simulink model "Clock_Model"  (R2025a)
settings: Solver=VariableStepAuto  StartTime=0.0  StopTime=1000  RelTol=1e-3
libraries: simulink_extras x27
(part 1 of 2)
settings Model: Creator=User  LastModifiedBy=User

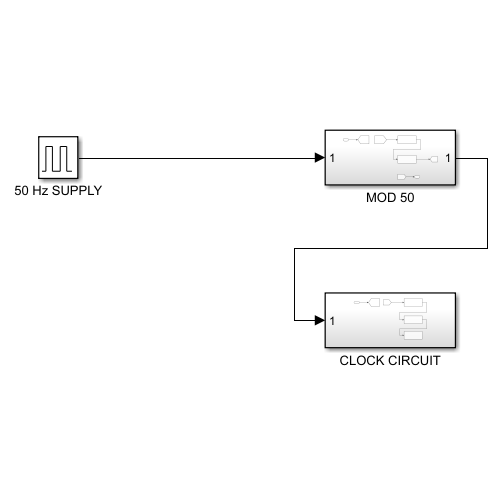
[thumbnail: Simulink's stored preview of the top-level diagram]
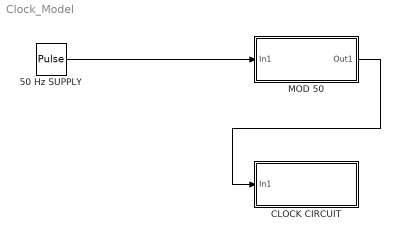
== system Clock_Model ==
  50 Hz SUPPLY : DiscretePulseGenerator  PulseType=Time based  Period=0.02  PulseWidth=50
  CLOCK CIRCUIT : Subsystem
  MOD 50 : Subsystem
  wires:
  50 Hz SUPPLY/1 -> MOD 50/1(In1)
  MOD 50/1(Out1) -> CLOCK CIRCUIT/1(In1)

== system Clock_Model/CLOCK CIRCUIT ==
  In1 : Inport
  HOURS : Subsystem
  MINUTES : Subsystem
  SECONDS : Subsystem
  wires:
  [Supply] -> SECONDS/1(In1)
  In1/1 -> [Supply]
  SECONDS/1(Out1) -> MINUTES/1(In2)
  MINUTES/1(Out1) -> HOURS/1(In1)

== system Clock_Model/MOD 50 ==
  In1 : Inport
  MOD 10 : Subsystem
  MOD 5 : Subsystem
  Out1 : Outport
  wires:
  In1/1 -> [Supply]
  MOD 10/1(Out1) -> MOD 5/1(In2)
  MOD 5/1(Out1) -> [Pulse]
  [Pulse] -> Out1/1
  [Supply] -> MOD 10/1(In1)

== system Clock_Model/CLOCK CIRCUIT/HOURS ==
  In1 : Inport
  MOD 13 : Subsystem
  wires:
  In1/1 -> MOD 13/1(In2)

== system Clock_Model/CLOCK CIRCUIT/MINUTES ==
  In2 : Inport
  MOD 60 : Subsystem
  Out1 : Outport
  wires:
  In2/1 -> MOD 60/1(In2)
  MOD 60/1(Out1) -> Out1/1

== system Clock_Model/CLOCK CIRCUIT/SECONDS ==
  In1 : Inport
  MOD 60 : Subsystem
  Out1 : Outport
  wires:
  In1/1 -> MOD 60/1(In2)
  MOD 60/1(Out1) -> Out1/1

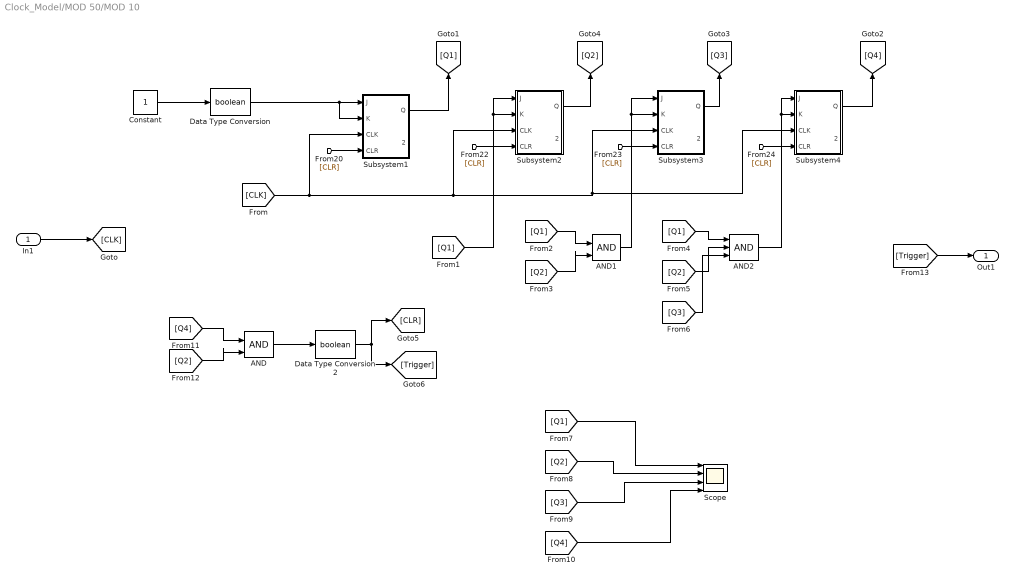
== system Clock_Model/MOD 50/MOD 10 ==
  In1 : Inport
  AND : Logic  IconShape=distinctive  AllPortsSameDT=off  OutDataTypeStr=boolean
  AND1 : Logic  IconShape=distinctive  AllPortsSameDT=off  OutDataTypeStr=boolean
  AND2 : Logic  Inputs=3  IconShape=distinctive  AllPortsSameDT=off  OutDataTypeStr=boolean
  Constant : Constant
  Data Type Conversion : DataTypeConversion  OutDataTypeStr=boolean  SaturateOnIntegerOverflow=off  RndMeth=Floor
  Data Type Conversion2 : DataTypeConversion  OutDataTypeStr=boolean  SaturateOnIntegerOverflow=off  RndMeth=Floor
  Scope : Scope  NumInputPorts=4
      settings: ActiveDisplayYMinimum=-1  ActiveDisplayYMaximum=1
  Subsystem1 : Subsystem
  Subsystem2 : Subsystem
  Subsystem3 : Subsystem
  Subsystem4 : Subsystem
  Out1 : Outport
  wires:
  [CLR] -> Subsystem2/4(CLR)
  [CLK] -> Subsystem1/3(CLK), Subsystem2/3(CLK), Subsystem4/3(CLK), Subsystem3/3(CLK)
  Data Type Conversion/1 -> Subsystem1/2(K), Subsystem1/1(J)
  [Q1] -> AND1/1
  AND1/1 -> Subsystem3/2(K), Subsystem3/1(J)
  [CLR] -> Subsystem1/4(CLR)
  [Q4] -> AND/1
  [Q2] -> AND2/2
  [Q1] -> AND2/1
  Subsystem1/1(Q) -> [Q1]
  [Q3] -> AND2/3
  [Q2] -> AND1/2
  Constant/1 -> Data Type Conversion/1
  AND2/1 -> Subsystem4/2(K), Subsystem4/1(J)
  Subsystem4/1(Q) -> [Q4]
  [CLR] -> Subsystem4/4(CLR)
  [Q1] -> Subsystem2/2(K), Subsystem2/1(J)
  [Q2] -> AND/2
  Subsystem2/1(Q) -> [Q2]
  Data Type Conversion2/1 -> [CLR], [Trigger]
  [CLR] -> Subsystem3/4(CLR)
  Subsystem3/1(Q) -> [Q3]
  AND/1 -> Data Type Conversion2/1
  In1/1 -> [CLK]
  [Trigger] -> Out1/1
  [Q1] -> Scope/1
  [Q2] -> Scope/2
  [Q3] -> Scope/3
  [Q4] -> Scope/4

== system Clock_Model/MOD 50/MOD 5 ==
  In2 : Inport
  AND : Logic  IconShape=distinctive  AllPortsSameDT=off  OutDataTypeStr=boolean
  AND1 : Logic  IconShape=distinctive  AllPortsSameDT=off  OutDataTypeStr=boolean
  Constant : Constant
  Data Type Conversion : DataTypeConversion  OutDataTypeStr=boolean  SaturateOnIntegerOverflow=off  RndMeth=Floor
  Data Type Conversion2 : DataTypeConversion  OutDataTypeStr=boolean  SaturateOnIntegerOverflow=off  RndMeth=Floor
  Scope : Scope  NumInputPorts=3
      settings: ActiveDisplayYMinimum=-1  ActiveDisplayYMaximum=1
  Subsystem1 : Subsystem
  Subsystem2 : Subsystem
  Subsystem3 : Subsystem
  Out1 : Outport
  wires:
  [Q3] -> AND/1
  AND1/1 -> Subsystem3/2(K), Subsystem3/1(J)
  Data Type Conversion/1 -> Subsystem1/2(K), Subsystem1/1(J)
  [Q1] -> AND1/1
  [CLR] -> Subsystem1/4(CLR)
  [CLK] -> Subsystem1/3(CLK), Subsystem2/3(CLK), Subsystem3/3(CLK)
  [CLR] -> Subsystem2/4(CLR)
  [Q1] -> Subsystem2/2(K), Subsystem2/1(J)
  Constant/1 -> Data Type Conversion/1
  [Q2] -> AND1/2
  Subsystem1/1(Q) -> [Q1]
  [CLR] -> Subsystem3/4(CLR)
  Subsystem2/1(Q) -> [Q2]
  [Q1] -> AND/2
  AND/1 -> Data Type Conversion2/1
  Subsystem3/1(Q) -> [Q3]
  Data Type Conversion2/1 -> [Trigger], [CLR]
  [Q1] -> Scope/1
  [Q2] -> Scope/2
  [Q3] -> Scope/3
  [Trigger] -> Out1/1
  In2/1 -> [CLK]

== system Clock_Model/CLOCK CIRCUIT/HOURS/MOD 13 ==
  In2 : Inport
  MOD 10 : Subsystem
  MOD 2 : Subsystem
  wires:
  In2/1 -> [Supply]
  MOD 10/1(Out1) -> MOD 2/1(In2)
  [Supply] -> MOD 10/1(In1)

== system Clock_Model/CLOCK CIRCUIT/MINUTES/MOD 60 ==
  In2 : Inport
  MOD 10 : Subsystem
  MOD 6 : Subsystem
  Out1 : Outport
  wires:
  [Supply] -> MOD 10/1(In1)
  In2/1 -> [Supply]
  MOD 10/1(Out1) -> MOD 6/1(In2)
  MOD 6/1(Out1) -> Out1/1

== system Clock_Model/CLOCK CIRCUIT/SECONDS/MOD 60 ==
  In2 : Inport
  MOD 10 : Subsystem
  MOD 6 : Subsystem
  Out1 : Outport
  wires:
  [Supply] -> MOD 10/1(In1)
  In2/1 -> [Supply]
  MOD 10/1(Out1) -> MOD 6/1(In2)
  MOD 6/1(Out1) -> Out1/1

== system Clock_Model/MOD 50/MOD 10/Subsystem1 ==
  J : Inport
  K : Inport  Port=2
  CLK : Inport  Port=3
  CLR : Inport  Port=4
  Constant : Constant  Value=0
  Constant1 : Constant
  Data Type Conversion : DataTypeConversion  OutDataTypeStr=double  SaturateOnIntegerOverflow=off  RndMeth=Floor
  Data Type Conversion{1,3..5} (4 alike) : DataTypeConversion  OutDataTypeStr=boolean  SaturateOnIntegerOverflow=off  RndMeth=Floor
  Data Type Conversion2 : DataTypeConversion  OutDataTypeStr=double  SaturateOnIntegerOverflow=off  RndMeth=Floor
  J-K Flip-Flop : simulink_extras/Flip Flops/J-K Flip-Flop  initial_condition=0
  Memory : Memory
  Switch : Switch  Criteria=u2 > Threshold  Threshold=0.5  SaturateOnIntegerOverflow=off  InputSameDT=off
  Switch1 : Switch  Criteria=u2 > Threshold  Threshold=0.5  SaturateOnIntegerOverflow=off  InputSameDT=off
  Q : Outport
  Q BAR : Outport  Port=2
  wires:
  J-K Flip-Flop/1 -> Data Type Conversion4/1
  J-K Flip-Flop/2 -> Data Type Conversion5/1
  J/1 -> Data Type Conversion/1
  CLR/1 -> Memory/1
  [CLR] -> Switch/2
  Switch/1 -> Data Type Conversion1/1
  Data Type Conversion1/1 -> J-K Flip-Flop/1
  CLK/1 -> J-K Flip-Flop/2
  Data Type Conversion3/1 -> J-K Flip-Flop/3
  Switch1/1 -> Data Type Conversion3/1
  [CLR] -> Switch1/2
  K/1 -> Data Type Conversion2/1
  Memory/1 -> [CLR]
  Constant/1 -> Switch/1
  Data Type Conversion/1 -> Switch/3
  Data Type Conversion4/1 -> Q/1
  Data Type Conversion5/1 -> Q BAR/1
  Constant1/1 -> Switch1/1
  Data Type Conversion2/1 -> Switch1/3

== system Clock_Model/MOD 50/MOD 10/Subsystem2 ==
  J : Inport
  K : Inport  Port=2
  CLK : Inport  Port=3
  CLR : Inport  Port=4
  Constant : Constant  Value=0
  Constant1 : Constant
  Data Type Conversion : DataTypeConversion  OutDataTypeStr=double  SaturateOnIntegerOverflow=off  RndMeth=Floor
  Data Type Conversion{1,3..5} (4 alike) : DataTypeConversion  OutDataTypeStr=boolean  SaturateOnIntegerOverflow=off  RndMeth=Floor
  Data Type Conversion2 : DataTypeConversion  OutDataTypeStr=double  SaturateOnIntegerOverflow=off  RndMeth=Floor
  J-K Flip-Flop : simulink_extras/Flip Flops/J-K Flip-Flop  initial_condition=0
  Switch : Switch  Criteria=u2 > Threshold  Threshold=0.5  SaturateOnIntegerOverflow=off  InputSameDT=off
  Switch1 : Switch  Criteria=u2 > Threshold  Threshold=0.5  SaturateOnIntegerOverflow=off  InputSameDT=off
  Q : Outport
  Q BAR : Outport  Port=2
  wires:
  J-K Flip-Flop/1 -> Data Type Conversion4/1
  J-K Flip-Flop/2 -> Data Type Conversion5/1
  J/1 -> Data Type Conversion/1
  CLR/1 -> [CLR]
  [CLR] -> Switch/2
  Switch/1 -> Data Type Conversion1/1
  Data Type Conversion1/1 -> J-K Flip-Flop/1
  CLK/1 -> J-K Flip-Flop/2
  Data Type Conversion3/1 -> J-K Flip-Flop/3
  Switch1/1 -> Data Type Conversion3/1
  [CLR] -> Switch1/2
  K/1 -> Data Type Conversion2/1
  Constant/1 -> Switch/1
  Data Type Conversion/1 -> Switch/3
  Data Type Conversion4/1 -> Q/1
  Data Type Conversion5/1 -> Q BAR/1
  Constant1/1 -> Switch1/1
  Data Type Conversion2/1 -> Switch1/3

== system Clock_Model/MOD 50/MOD 10/Subsystem3 ==
  J : Inport
  K : Inport  Port=2
  CLK : Inport  Port=3
  CLR : Inport  Port=4
  Constant : Constant  Value=0
  Constant1 : Constant
  Data Type Conversion : DataTypeConversion  OutDataTypeStr=double  SaturateOnIntegerOverflow=off  RndMeth=Floor
  Data Type Conversion{1,3..5} (4 alike) : DataTypeConversion  OutDataTypeStr=boolean  SaturateOnIntegerOverflow=off  RndMeth=Floor
  Data Type Conversion2 : DataTypeConversion  OutDataTypeStr=double  SaturateOnIntegerOverflow=off  RndMeth=Floor
  J-K Flip-Flop : simulink_extras/Flip Flops/J-K Flip-Flop  initial_condition=0
  Switch : Switch  Criteria=u2 > Threshold  Threshold=0.5  SaturateOnIntegerOverflow=off  InputSameDT=off
  Switch1 : Switch  Criteria=u2 > Threshold  Threshold=0.5  SaturateOnIntegerOverflow=off  InputSameDT=off
  Q : Outport
  Q BAR : Outport  Port=2
  wires:
  J-K Flip-Flop/1 -> Data Type Conversion4/1
  J-K Flip-Flop/2 -> Data Type Conversion5/1
  J/1 -> Data Type Conversion/1
  CLR/1 -> [CLR]
  [CLR] -> Switch/2
  Switch/1 -> Data Type Conversion1/1
  Data Type Conversion1/1 -> J-K Flip-Flop/1
  CLK/1 -> J-K Flip-Flop/2
  Data Type Conversion3/1 -> J-K Flip-Flop/3
  Switch1/1 -> Data Type Conversion3/1
  [CLR] -> Switch1/2
  K/1 -> Data Type Conversion2/1
  Constant/1 -> Switch/1
  Data Type Conversion/1 -> Switch/3
  Data Type Conversion4/1 -> Q/1
  Data Type Conversion5/1 -> Q BAR/1
  Data Type Conversion2/1 -> Switch1/3
  Constant1/1 -> Switch1/1

== system Clock_Model/MOD 50/MOD 10/Subsystem4 ==
  J : Inport
  K : Inport  Port=2
  CLK : Inport  Port=3
  CLR : Inport  Port=4
  Constant : Constant  Value=0
  Constant1 : Constant
  Data Type Conversion : DataTypeConversion  OutDataTypeStr=double  SaturateOnIntegerOverflow=off  RndMeth=Floor
  Data Type Conversion{1,3..5} (4 alike) : DataTypeConversion  OutDataTypeStr=boolean  SaturateOnIntegerOverflow=off  RndMeth=Floor
  Data Type Conversion2 : DataTypeConversion  OutDataTypeStr=double  SaturateOnIntegerOverflow=off  RndMeth=Floor
  J-K Flip-Flop : simulink_extras/Flip Flops/J-K Flip-Flop  initial_condition=0
  Switch : Switch  Criteria=u2 > Threshold  Threshold=0.5  SaturateOnIntegerOverflow=off  InputSameDT=off
  Switch1 : Switch  Criteria=u2 > Threshold  Threshold=0.5  SaturateOnIntegerOverflow=off  InputSameDT=off
  Q : Outport
  Q BAR : Outport  Port=2
  wires:
  J-K Flip-Flop/1 -> Data Type Conversion4/1
  J-K Flip-Flop/2 -> Data Type Conversion5/1
  J/1 -> Data Type Conversion/1
  CLR/1 -> [CLR]
  [CLR] -> Switch/2
  Switch/1 -> Data Type Conversion1/1
  Data Type Conversion1/1 -> J-K Flip-Flop/1
  CLK/1 -> J-K Flip-Flop/2
  Data Type Conversion3/1 -> J-K Flip-Flop/3
  Switch1/1 -> Data Type Conversion3/1
  [CLR] -> Switch1/2
  K/1 -> Data Type Conversion2/1
  Data Type Conversion/1 -> Switch/3
  Constant/1 -> Switch/1
  Data Type Conversion4/1 -> Q/1
  Data Type Conversion5/1 -> Q BAR/1
  Constant1/1 -> Switch1/1
  Data Type Conversion2/1 -> Switch1/3

== system Clock_Model/MOD 50/MOD 5/Subsystem1 ==
  J : Inport
  K : Inport  Port=2
  CLK : Inport  Port=3
  CLR : Inport  Port=4
  Constant : Constant  Value=0
  Constant1 : Constant
  Data Type Conversion : DataTypeConversion  OutDataTypeStr=double  SaturateOnIntegerOverflow=off  RndMeth=Floor
  Data Type Conversion{1,3..5} (4 alike) : DataTypeConversion  OutDataTypeStr=boolean  SaturateOnIntegerOverflow=off  RndMeth=Floor
  Data Type Conversion2 : DataTypeConversion  OutDataTypeStr=double  SaturateOnIntegerOverflow=off  RndMeth=Floor
  J-K Flip-Flop : simulink_extras/Flip Flops/J-K Flip-Flop  initial_condition=0
  Memory : Memory
  Switch : Switch  Criteria=u2 > Threshold  Threshold=0.5  SaturateOnIntegerOverflow=off  InputSameDT=off
  Switch1 : Switch  Criteria=u2 > Threshold  Threshold=0.5  SaturateOnIntegerOverflow=off  InputSameDT=off
  Q : Outport
  Q BAR : Outport  Port=2
  wires:
  J-K Flip-Flop/1 -> Data Type Conversion4/1
  J-K Flip-Flop/2 -> Data Type Conversion5/1
  J/1 -> Data Type Conversion/1
  CLR/1 -> Memory/1
  [CLR] -> Switch/2
  Switch/1 -> Data Type Conversion1/1
  Data Type Conversion1/1 -> J-K Flip-Flop/1
  CLK/1 -> J-K Flip-Flop/2
  Data Type Conversion3/1 -> J-K Flip-Flop/3
  Switch1/1 -> Data Type Conversion3/1
  [CLR] -> Switch1/2
  K/1 -> Data Type Conversion2/1
  Memory/1 -> [CLR]
  Constant/1 -> Switch/1
  Data Type Conversion/1 -> Switch/3
  Data Type Conversion4/1 -> Q/1
  Data Type Conversion5/1 -> Q BAR/1
  Constant1/1 -> Switch1/1
  Data Type Conversion2/1 -> Switch1/3

== system Clock_Model/MOD 50/MOD 5/Subsystem2 ==
  J : Inport
  K : Inport  Port=2
  CLK : Inport  Port=3
  CLR : Inport  Port=4
  Constant : Constant  Value=0
  Constant1 : Constant
  Data Type Conversion : DataTypeConversion  OutDataTypeStr=double  SaturateOnIntegerOverflow=off  RndMeth=Floor
  Data Type Conversion{1,3..5} (4 alike) : DataTypeConversion  OutDataTypeStr=boolean  SaturateOnIntegerOverflow=off  RndMeth=Floor
  Data Type Conversion2 : DataTypeConversion  OutDataTypeStr=double  SaturateOnIntegerOverflow=off  RndMeth=Floor
  J-K Flip-Flop : simulink_extras/Flip Flops/J-K Flip-Flop  initial_condition=0
  Switch : Switch  Criteria=u2 > Threshold  Threshold=0.5  SaturateOnIntegerOverflow=off  InputSameDT=off
  Switch1 : Switch  Criteria=u2 > Threshold  Threshold=0.5  SaturateOnIntegerOverflow=off  InputSameDT=off
  Q : Outport
  Q BAR : Outport  Port=2
  wires:
  J-K Flip-Flop/1 -> Data Type Conversion4/1
  J-K Flip-Flop/2 -> Data Type Conversion5/1
  J/1 -> Data Type Conversion/1
  CLR/1 -> [CLR]
  [CLR] -> Switch/2
  Switch/1 -> Data Type Conversion1/1
  Data Type Conversion1/1 -> J-K Flip-Flop/1
  CLK/1 -> J-K Flip-Flop/2
  Data Type Conversion3/1 -> J-K Flip-Flop/3
  Switch1/1 -> Data Type Conversion3/1
  [CLR] -> Switch1/2
  K/1 -> Data Type Conversion2/1
  Constant/1 -> Switch/1
  Data Type Conversion/1 -> Switch/3
  Data Type Conversion4/1 -> Q/1
  Data Type Conversion5/1 -> Q BAR/1
  Constant1/1 -> Switch1/1
  Data Type Conversion2/1 -> Switch1/3

== system Clock_Model/MOD 50/MOD 5/Subsystem3 ==
  J : Inport
  K : Inport  Port=2
  CLK : Inport  Port=3
  CLR : Inport  Port=4
  Constant : Constant  Value=0
  Constant1 : Constant
  Data Type Conversion : DataTypeConversion  OutDataTypeStr=double  SaturateOnIntegerOverflow=off  RndMeth=Floor
  Data Type Conversion{1,3..5} (4 alike) : DataTypeConversion  OutDataTypeStr=boolean  SaturateOnIntegerOverflow=off  RndMeth=Floor
  Data Type Conversion2 : DataTypeConversion  OutDataTypeStr=double  SaturateOnIntegerOverflow=off  RndMeth=Floor
  J-K Flip-Flop : simulink_extras/Flip Flops/J-K Flip-Flop  initial_condition=0
  Switch : Switch  Criteria=u2 > Threshold  Threshold=0.5  SaturateOnIntegerOverflow=off  InputSameDT=off
  Switch1 : Switch  Criteria=u2 > Threshold  Threshold=0.5  SaturateOnIntegerOverflow=off  InputSameDT=off
  Q : Outport
  Q BAR : Outport  Port=2
  wires:
  J-K Flip-Flop/1 -> Data Type Conversion4/1
  J-K Flip-Flop/2 -> Data Type Conversion5/1
  J/1 -> Data Type Conversion/1
  CLR/1 -> [CLR]
  [CLR] -> Switch/2
  Switch/1 -> Data Type Conversion1/1
  Data Type Conversion1/1 -> J-K Flip-Flop/1
  CLK/1 -> J-K Flip-Flop/2
  Data Type Conversion3/1 -> J-K Flip-Flop/3
  Switch1/1 -> Data Type Conversion3/1
  [CLR] -> Switch1/2
  K/1 -> Data Type Conversion2/1
  Constant/1 -> Switch/1
  Data Type Conversion/1 -> Switch/3
  Data Type Conversion4/1 -> Q/1
  Data Type Conversion5/1 -> Q BAR/1
  Data Type Conversion2/1 -> Switch1/3
  Constant1/1 -> Switch1/1

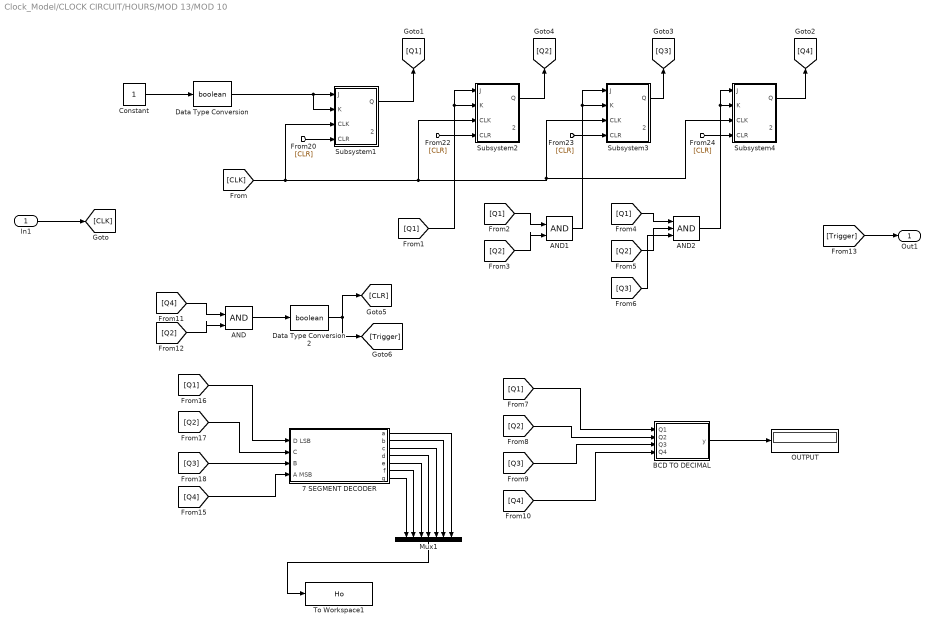
== system Clock_Model/CLOCK CIRCUIT/HOURS/MOD 13/MOD 10 ==
  In1 : Inport
  7 SEGMENT DECODER : Subsystem
  AND : Logic  IconShape=distinctive  AllPortsSameDT=off  OutDataTypeStr=boolean
  AND1 : Logic  IconShape=distinctive  AllPortsSameDT=off  OutDataTypeStr=boolean
  AND2 : Logic  Inputs=3  IconShape=distinctive  AllPortsSameDT=off  OutDataTypeStr=boolean
  BCD TO DECIMAL : MATLAB Function  TreatAsAtomicUnit=on
  Constant : Constant
  Data Type Conversion : DataTypeConversion  OutDataTypeStr=boolean  SaturateOnIntegerOverflow=off  RndMeth=Floor
  Data Type Conversion2 : DataTypeConversion  OutDataTypeStr=boolean  SaturateOnIntegerOverflow=off  RndMeth=Floor
  Mux1 : Mux  Inputs=7
  OUTPUT : Display
  Subsystem1 : Subsystem
  Subsystem2 : Subsystem
  Subsystem3 : Subsystem
  Subsystem4 : Subsystem
  To Workspace1 : ToWorkspace  VariableName=Ho  SampleTime=-1
  Out1 : Outport
  wires:
  [CLR] -> Subsystem2/4(CLR)
  [CLK] -> Subsystem1/3(CLK), Subsystem2/3(CLK), Subsystem4/3(CLK), Subsystem3/3(CLK)
  Data Type Conversion/1 -> Subsystem1/2(K), Subsystem1/1(J)
  [Q1] -> AND1/1
  AND1/1 -> Subsystem3/2(K), Subsystem3/1(J)
  [CLR] -> Subsystem1/4(CLR)
  [Q4] -> AND/1
  [Q2] -> AND2/2
  [Q1] -> AND2/1
  Subsystem1/1(Q) -> [Q1]
  [Q3] -> AND2/3
  [Q2] -> AND1/2
  Constant/1 -> Data Type Conversion/1
  AND2/1 -> Subsystem4/2(K), Subsystem4/1(J)
  Subsystem4/1(Q) -> [Q4]
  [CLR] -> Subsystem4/4(CLR)
  [Q1] -> Subsystem2/2(K), Subsystem2/1(J)
  [Q2] -> AND/2
  Subsystem2/1(Q) -> [Q2]
  Data Type Conversion2/1 -> [CLR], [Trigger]
  [CLR] -> Subsystem3/4(CLR)
  Subsystem3/1(Q) -> [Q3]
  AND/1 -> Data Type Conversion2/1
  In1/1 -> [CLK]
  [Trigger] -> Out1/1
  [Q1] -> BCD TO DECIMAL/1(Q1)
  [Q2] -> BCD TO DECIMAL/2(Q2)
  [Q3] -> BCD TO DECIMAL/3(Q3)
  [Q4] -> BCD TO DECIMAL/4(Q4)
  BCD TO DECIMAL/1(y) -> OUTPUT/1
  7 SEGMENT DECODER/7(g) -> Mux1/1
  7 SEGMENT DECODER/6(f) -> Mux1/2
  [Q4] -> 7 SEGMENT DECODER/4(A MSB)
  [Q3] -> 7 SEGMENT DECODER/3(B)
  7 SEGMENT DECODER/1(a) -> Mux1/7
  7 SEGMENT DECODER/4(d) -> Mux1/4
  Mux1/1 -> To Workspace1/1
  7 SEGMENT DECODER/5(e) -> Mux1/3
  [Q1] -> 7 SEGMENT DECODER/1(D LSB)
  [Q2] -> 7 SEGMENT DECODER/2(C)
  7 SEGMENT DECODER/3(c) -> Mux1/5
  7 SEGMENT DECODER/2(b) -> Mux1/6

== system Clock_Model/CLOCK CIRCUIT/HOURS/MOD 13/MOD 2 ==
  In2 : Inport
  7 SEGMENT DECODER : Subsystem
  AND : Logic  IconShape=distinctive  AllPortsSameDT=off  OutDataTypeStr=boolean
  Constant : Constant
  Constant1 : Constant  Value=0
  Constant2 : Constant  Value=0
  Data Type Conversion{,1..3} (4 alike) : DataTypeConversion  OutDataTypeStr=boolean  SaturateOnIntegerOverflow=off  RndMeth=Floor
  Mux1 : Mux  Inputs=7
  NOT : Logic  Operator=NOT  IconShape=distinctive  AllPortsSameDT=off  OutDataTypeStr=boolean
  Subsystem1 : Subsystem
  Subsystem2 : Subsystem
  To Workspace1 : ToWorkspace  VariableName=Ht  SampleTime=-1
  wires:
  In2/1 -> [CLK]
  [Q2] -> AND/1
  Data Type Conversion/1 -> Subsystem1/2(K), Subsystem1/1(J)
  [CLR] -> Subsystem1/4(CLR)
  [CLK] -> Subsystem1/3(CLK), Subsystem2/3(CLK)
  [CLR] -> Subsystem2/4(CLR)
  [Q1] -> Subsystem2/2(K), Subsystem2/1(J)
  Constant/1 -> Data Type Conversion/1
  Subsystem1/1(Q) -> [Q1]
  Subsystem2/1(Q) -> [Q2]
  [Q1] -> NOT/1
  AND/1 -> Data Type Conversion2/1
  Data Type Conversion2/1 -> [CLR]
  7 SEGMENT DECODER/7(g) -> Mux1/1
  7 SEGMENT DECODER/6(f) -> Mux1/2
  Data Type Conversion1/1 -> 7 SEGMENT DECODER/4(A MSB)
  Data Type Conversion3/1 -> 7 SEGMENT DECODER/3(B)
  7 SEGMENT DECODER/1(a) -> Mux1/7
  7 SEGMENT DECODER/4(d) -> Mux1/4
  Mux1/1 -> To Workspace1/1
  7 SEGMENT DECODER/5(e) -> Mux1/3
  [Q1] -> 7 SEGMENT DECODER/1(D LSB)
  [Q2] -> 7 SEGMENT DECODER/2(C)
  7 SEGMENT DECODER/3(c) -> Mux1/5
  7 SEGMENT DECODER/2(b) -> Mux1/6
  Constant1/1 -> Data Type Conversion1/1
  Constant2/1 -> Data Type Conversion3/1
  NOT/1 -> AND/2

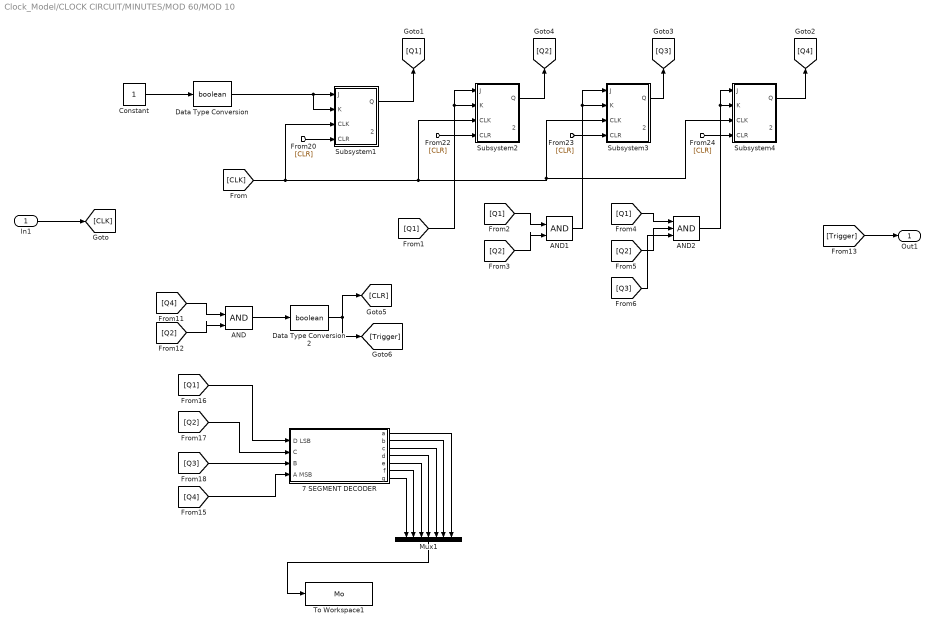
== system Clock_Model/CLOCK CIRCUIT/MINUTES/MOD 60/MOD 10 ==
  In1 : Inport
  7 SEGMENT DECODER : Subsystem
  AND : Logic  IconShape=distinctive  AllPortsSameDT=off  OutDataTypeStr=boolean
  AND1 : Logic  IconShape=distinctive  AllPortsSameDT=off  OutDataTypeStr=boolean
  AND2 : Logic  Inputs=3  IconShape=distinctive  AllPortsSameDT=off  OutDataTypeStr=boolean
  Constant : Constant
  Data Type Conversion : DataTypeConversion  OutDataTypeStr=boolean  SaturateOnIntegerOverflow=off  RndMeth=Floor
  Data Type Conversion2 : DataTypeConversion  OutDataTypeStr=boolean  SaturateOnIntegerOverflow=off  RndMeth=Floor
  Mux1 : Mux  Inputs=7
  Subsystem1 : Subsystem
  Subsystem2 : Subsystem
  Subsystem3 : Subsystem
  Subsystem4 : Subsystem
  To Workspace1 : ToWorkspace  VariableName=Mo  SampleTime=-1
  Out1 : Outport
  wires:
  [CLR] -> Subsystem2/4(CLR)
  [CLK] -> Subsystem1/3(CLK), Subsystem2/3(CLK), Subsystem4/3(CLK), Subsystem3/3(CLK)
  Data Type Conversion/1 -> Subsystem1/2(K), Subsystem1/1(J)
  [Q1] -> AND1/1
  AND1/1 -> Subsystem3/2(K), Subsystem3/1(J)
  [CLR] -> Subsystem1/4(CLR)
  [Q4] -> AND/1
  [Q2] -> AND2/2
  [Q1] -> AND2/1
  Subsystem1/1(Q) -> [Q1]
  [Q3] -> AND2/3
  [Q2] -> AND1/2
  Constant/1 -> Data Type Conversion/1
  AND2/1 -> Subsystem4/2(K), Subsystem4/1(J)
  Subsystem4/1(Q) -> [Q4]
  [CLR] -> Subsystem4/4(CLR)
  [Q1] -> Subsystem2/2(K), Subsystem2/1(J)
  [Q2] -> AND/2
  Subsystem2/1(Q) -> [Q2]
  Data Type Conversion2/1 -> [CLR], [Trigger]
  [CLR] -> Subsystem3/4(CLR)
  Subsystem3/1(Q) -> [Q3]
  AND/1 -> Data Type Conversion2/1
  In1/1 -> [CLK]
  [Trigger] -> Out1/1
  7 SEGMENT DECODER/7(g) -> Mux1/1
  7 SEGMENT DECODER/6(f) -> Mux1/2
  [Q4] -> 7 SEGMENT DECODER/4(A MSB)
  [Q3] -> 7 SEGMENT DECODER/3(B)
  7 SEGMENT DECODER/1(a) -> Mux1/7
  7 SEGMENT DECODER/4(d) -> Mux1/4
  Mux1/1 -> To Workspace1/1
  7 SEGMENT DECODER/5(e) -> Mux1/3
  [Q1] -> 7 SEGMENT DECODER/1(D LSB)
  [Q2] -> 7 SEGMENT DECODER/2(C)
  7 SEGMENT DECODER/3(c) -> Mux1/5
  7 SEGMENT DECODER/2(b) -> Mux1/6

== system Clock_Model/CLOCK CIRCUIT/MINUTES/MOD 60/MOD 6 ==
  In2 : Inport
  7 SEGMENT DECODER : Subsystem
  AND : Logic  IconShape=distinctive  AllPortsSameDT=off  OutDataTypeStr=boolean
  AND1 : Logic  IconShape=distinctive  AllPortsSameDT=off  OutDataTypeStr=boolean
  Constant : Constant
  Constant1 : Constant  Value=0
  Data Type Conversion : DataTypeConversion  OutDataTypeStr=boolean  SaturateOnIntegerOverflow=off  RndMeth=Floor
  Data Type Conversion1 : DataTypeConversion  OutDataTypeStr=boolean  SaturateOnIntegerOverflow=off  RndMeth=Floor
  Data Type Conversion2 : DataTypeConversion  OutDataTypeStr=boolean  SaturateOnIntegerOverflow=off  RndMeth=Floor
  Mux1 : Mux  Inputs=7
  Subsystem1 : Subsystem
  Subsystem2 : Subsystem
  Subsystem3 : Subsystem
  To Workspace1 : ToWorkspace  VariableName=Mt  SampleTime=-1
  Out1 : Outport
  wires:
  In2/1 -> [CLK]
  [Q3] -> AND/1
  AND1/1 -> Subsystem3/2(K), Subsystem3/1(J)
  Data Type Conversion/1 -> Subsystem1/2(K), Subsystem1/1(J)
  [Q1] -> AND1/1
  [CLR] -> Subsystem1/4(CLR)
  [CLK] -> Subsystem1/3(CLK), Subsystem2/3(CLK), Subsystem3/3(CLK)
  [CLR] -> Subsystem2/4(CLR)
  [Q1] -> Subsystem2/2(K), Subsystem2/1(J)
  Constant/1 -> Data Type Conversion/1
  [Q2] -> AND1/2
  Subsystem1/1(Q) -> [Q1]
  [CLR] -> Subsystem3/4(CLR)
  Subsystem2/1(Q) -> [Q2]
  [Q2] -> AND/2
  AND/1 -> Data Type Conversion2/1
  Subsystem3/1(Q) -> [Q3]
  Data Type Conversion2/1 -> Out1/1, [CLR]
  7 SEGMENT DECODER/7(g) -> Mux1/1
  7 SEGMENT DECODER/6(f) -> Mux1/2
  Data Type Conversion1/1 -> 7 SEGMENT DECODER/4(A MSB)
  [Q3] -> 7 SEGMENT DECODER/3(B)
  7 SEGMENT DECODER/1(a) -> Mux1/7
  7 SEGMENT DECODER/4(d) -> Mux1/4
  Mux1/1 -> To Workspace1/1
  7 SEGMENT DECODER/5(e) -> Mux1/3
  [Q1] -> 7 SEGMENT DECODER/1(D LSB)
  [Q2] -> 7 SEGMENT DECODER/2(C)
  7 SEGMENT DECODER/3(c) -> Mux1/5
  7 SEGMENT DECODER/2(b) -> Mux1/6
  Constant1/1 -> Data Type Conversion1/1

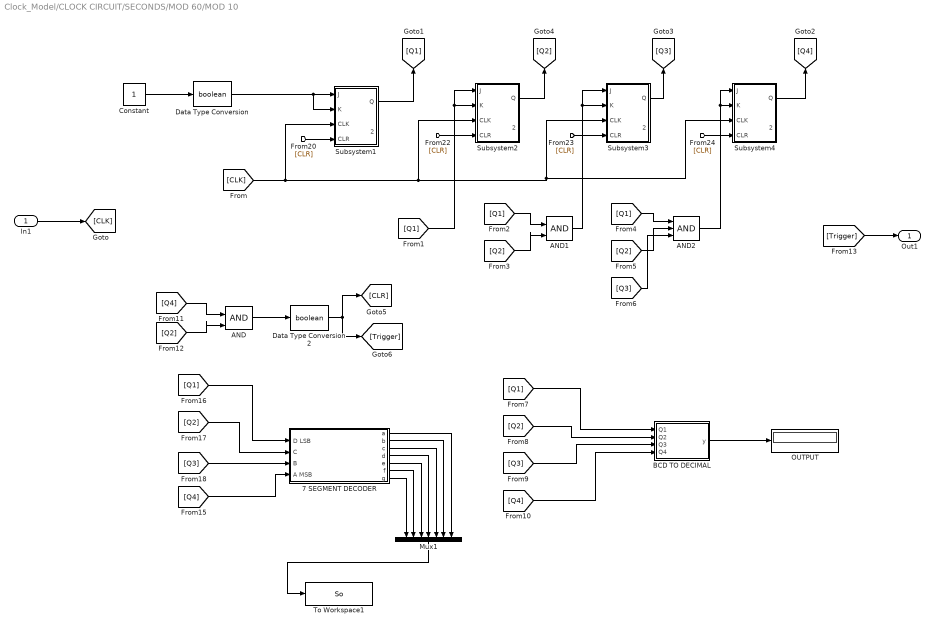
== system Clock_Model/CLOCK CIRCUIT/SECONDS/MOD 60/MOD 10 ==
  In1 : Inport
  7 SEGMENT DECODER : Subsystem
  AND : Logic  IconShape=distinctive  AllPortsSameDT=off  OutDataTypeStr=boolean
  AND1 : Logic  IconShape=distinctive  AllPortsSameDT=off  OutDataTypeStr=boolean
  AND2 : Logic  Inputs=3  IconShape=distinctive  AllPortsSameDT=off  OutDataTypeStr=boolean
  BCD TO DECIMAL : MATLAB Function  TreatAsAtomicUnit=on
  Constant : Constant
  Data Type Conversion : DataTypeConversion  OutDataTypeStr=boolean  SaturateOnIntegerOverflow=off  RndMeth=Floor
  Data Type Conversion2 : DataTypeConversion  OutDataTypeStr=boolean  SaturateOnIntegerOverflow=off  RndMeth=Floor
  Mux1 : Mux  Inputs=7
  OUTPUT : Display
  Subsystem1 : Subsystem
  Subsystem2 : Subsystem
  Subsystem3 : Subsystem
  Subsystem4 : Subsystem
  To Workspace1 : ToWorkspace  VariableName=So  SampleTime=-1
  Out1 : Outport
  wires:
  [CLR] -> Subsystem2/4(CLR)
  [CLK] -> Subsystem1/3(CLK), Subsystem2/3(CLK), Subsystem4/3(CLK), Subsystem3/3(CLK)
  Data Type Conversion/1 -> Subsystem1/2(K), Subsystem1/1(J)
  [Q1] -> AND1/1
  AND1/1 -> Subsystem3/2(K), Subsystem3/1(J)
  [CLR] -> Subsystem1/4(CLR)
  [Q4] -> AND/1
  [Q2] -> AND2/2
  [Q1] -> AND2/1
  Subsystem1/1(Q) -> [Q1]
  [Q3] -> AND2/3
  [Q2] -> AND1/2
  Constant/1 -> Data Type Conversion/1
  AND2/1 -> Subsystem4/2(K), Subsystem4/1(J)
  Subsystem4/1(Q) -> [Q4]
  [CLR] -> Subsystem4/4(CLR)
  [Q1] -> Subsystem2/2(K), Subsystem2/1(J)
  [Q2] -> AND/2
  Subsystem2/1(Q) -> [Q2]
  Data Type Conversion2/1 -> [CLR], [Trigger]
  [CLR] -> Subsystem3/4(CLR)
  Subsystem3/1(Q) -> [Q3]
  AND/1 -> Data Type Conversion2/1
  In1/1 -> [CLK]
  [Trigger] -> Out1/1
  [Q1] -> BCD TO DECIMAL/1(Q1)
  [Q2] -> BCD TO DECIMAL/2(Q2)
  [Q3] -> BCD TO DECIMAL/3(Q3)
  [Q4] -> BCD TO DECIMAL/4(Q4)
  BCD TO DECIMAL/1(y) -> OUTPUT/1
  7 SEGMENT DECODER/7(g) -> Mux1/1
  7 SEGMENT DECODER/6(f) -> Mux1/2
  [Q4] -> 7 SEGMENT DECODER/4(A MSB)
  [Q3] -> 7 SEGMENT DECODER/3(B)
  7 SEGMENT DECODER/1(a) -> Mux1/7
  7 SEGMENT DECODER/4(d) -> Mux1/4
  Mux1/1 -> To Workspace1/1
  7 SEGMENT DECODER/5(e) -> Mux1/3
  [Q1] -> 7 SEGMENT DECODER/1(D LSB)
  [Q2] -> 7 SEGMENT DECODER/2(C)
  7 SEGMENT DECODER/3(c) -> Mux1/5
  7 SEGMENT DECODER/2(b) -> Mux1/6

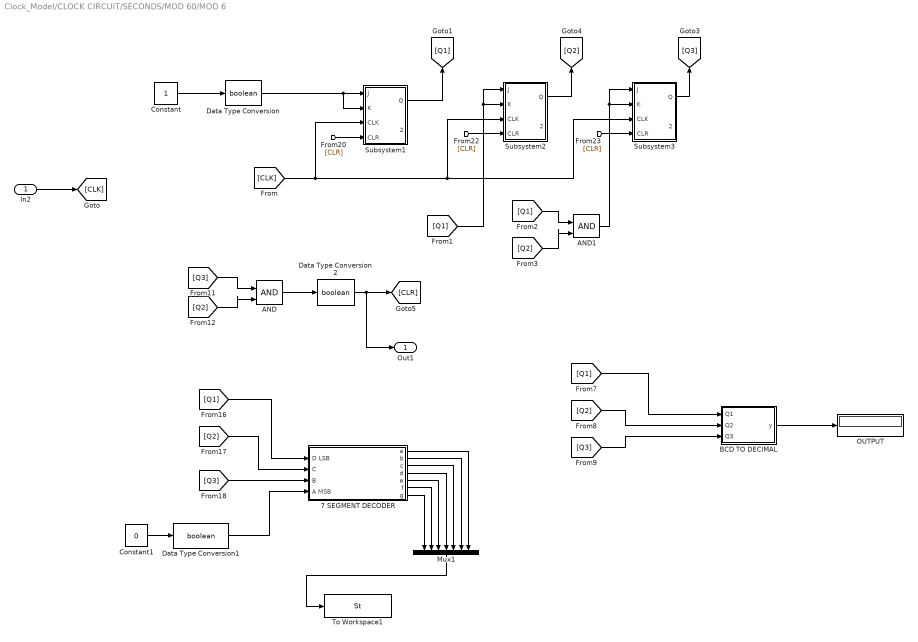
== system Clock_Model/CLOCK CIRCUIT/SECONDS/MOD 60/MOD 6 ==
  In2 : Inport
  7 SEGMENT DECODER : Subsystem
  AND : Logic  IconShape=distinctive  AllPortsSameDT=off  OutDataTypeStr=boolean
  AND1 : Logic  IconShape=distinctive  AllPortsSameDT=off  OutDataTypeStr=boolean
  BCD TO DECIMAL : MATLAB Function  TreatAsAtomicUnit=on
  Constant : Constant
  Constant1 : Constant  Value=0
  Data Type Conversion : DataTypeConversion  OutDataTypeStr=boolean  SaturateOnIntegerOverflow=off  RndMeth=Floor
  Data Type Conversion1 : DataTypeConversion  OutDataTypeStr=boolean  SaturateOnIntegerOverflow=off  RndMeth=Floor
  Data Type Conversion2 : DataTypeConversion  OutDataTypeStr=boolean  SaturateOnIntegerOverflow=off  RndMeth=Floor
  Mux1 : Mux  Inputs=7
  OUTPUT : Display
  Subsystem1 : Subsystem
  Subsystem2 : Subsystem
  Subsystem3 : Subsystem
  To Workspace1 : ToWorkspace  VariableName=St  SampleTime=-1
  Out1 : Outport
  wires:
  In2/1 -> [CLK]
  [Q3] -> AND/1
  AND1/1 -> Subsystem3/2(K), Subsystem3/1(J)
  Data Type Conversion/1 -> Subsystem1/2(K), Subsystem1/1(J)
  [Q1] -> AND1/1
  [CLR] -> Subsystem1/4(CLR)
  [CLK] -> Subsystem1/3(CLK), Subsystem2/3(CLK), Subsystem3/3(CLK)
  [CLR] -> Subsystem2/4(CLR)
  [Q1] -> Subsystem2/2(K), Subsystem2/1(J)
  Constant/1 -> Data Type Conversion/1
  [Q2] -> AND1/2
  Subsystem1/1(Q) -> [Q1]
  [CLR] -> Subsystem3/4(CLR)
  Subsystem2/1(Q) -> [Q2]
  [Q2] -> AND/2
  AND/1 -> Data Type Conversion2/1
  Subsystem3/1(Q) -> [Q3]
  Data Type Conversion2/1 -> Out1/1, [CLR]
  [Q3] -> BCD TO DECIMAL/3(Q3)
  [Q1] -> BCD TO DECIMAL/1(Q1)
  [Q2] -> BCD TO DECIMAL/2(Q2)
  BCD TO DECIMAL/1(y) -> OUTPUT/1
  7 SEGMENT DECODER/7(g) -> Mux1/1
  7 SEGMENT DECODER/6(f) -> Mux1/2
  Data Type Conversion1/1 -> 7 SEGMENT DECODER/4(A MSB)
  [Q3] -> 7 SEGMENT DECODER/3(B)
  7 SEGMENT DECODER/1(a) -> Mux1/7
  7 SEGMENT DECODER/4(d) -> Mux1/4
  Mux1/1 -> To Workspace1/1
  7 SEGMENT DECODER/5(e) -> Mux1/3
  [Q1] -> 7 SEGMENT DECODER/1(D LSB)
  [Q2] -> 7 SEGMENT DECODER/2(C)
  7 SEGMENT DECODER/3(c) -> Mux1/5
  7 SEGMENT DECODER/2(b) -> Mux1/6
  Constant1/1 -> Data Type Conversion1/1

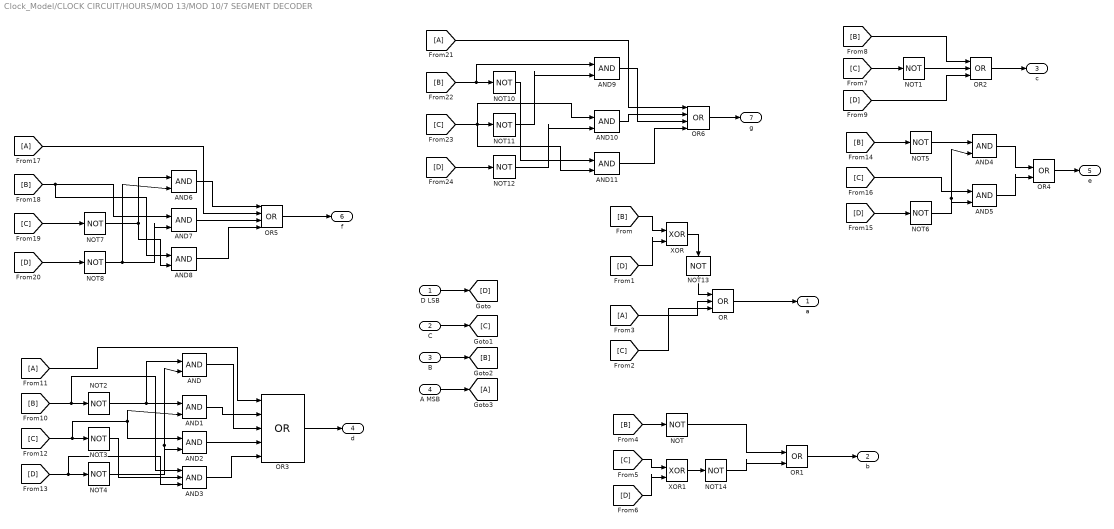
== system Clock_Model/CLOCK CIRCUIT/HOURS/MOD 13/MOD 10/7 SEGMENT DECODER ==
  D LSB : Inport
  C : Inport  Port=2
  B : Inport  Port=3
  A MSB : Inport  Port=4
  AND{,1..2,4..11} (11 alike) : Logic  IconShape=distinctive  AllPortsSameDT=off  OutDataTypeStr=boolean
  AND3 : Logic  Inputs=3  IconShape=distinctive  AllPortsSameDT=off  OutDataTypeStr=boolean
  From{3,11,17,21} (4 alike) : From
  Goto3 : Goto
  NOT{,1..8,10..14} (14 alike) : Logic  Operator=NOT  IconShape=distinctive  AllPortsSameDT=off  OutDataTypeStr=boolean
  OR : Logic  Operator=OR  Inputs=3  IconShape=distinctive  AllPortsSameDT=off  OutDataTypeStr=boolean
  OR1 : Logic  Operator=OR  IconShape=distinctive  AllPortsSameDT=off  OutDataTypeStr=boolean
  OR2 : Logic  Operator=OR  Inputs=3  IconShape=distinctive  AllPortsSameDT=off  OutDataTypeStr=boolean
  OR3 : Logic  Operator=OR  Inputs=5  IconShape=distinctive  AllPortsSameDT=off  OutDataTypeStr=boolean
  OR4 : Logic  Operator=OR  IconShape=distinctive  AllPortsSameDT=off  OutDataTypeStr=boolean
  OR5 : Logic  Operator=OR  Inputs=4  IconShape=distinctive  AllPortsSameDT=off  OutDataTypeStr=boolean
  OR6 : Logic  Operator=OR  Inputs=4  IconShape=distinctive  AllPortsSameDT=off  OutDataTypeStr=boolean
  XOR : Logic  Operator=XOR  IconShape=distinctive  AllPortsSameDT=off  OutDataTypeStr=boolean
  XOR1 : Logic  Operator=XOR  IconShape=distinctive  AllPortsSameDT=off  OutDataTypeStr=boolean
  a : Outport
  b : Outport  Port=2
  c : Outport  Port=3
  d : Outport  Port=4
  e : Outport  Port=5
  f : Outport  Port=6
  g : Outport  Port=7
  wires:
  D LSB/1 -> [D]
  C/1 -> [C]
  B/1 -> [B]
  A MSB/1 -> Goto3/1
  XOR/1 -> NOT13/1
  [B] -> XOR/1
  [D] -> XOR/2
  From3/1 -> OR/2
  [C] -> OR/3
  OR/1 -> a/1
  [B] -> NOT/1
  [C] -> XOR1/1
  [D] -> XOR1/2
  NOT/1 -> OR1/1
  XOR1/1 -> NOT14/1
  OR1/1 -> b/1
  [C] -> NOT1/1
  [B] -> OR2/1
  NOT1/1 -> OR2/2
  [D] -> OR2/3
  OR2/1 -> c/1
  [B] -> AND3/1, NOT2/1
  [C] -> AND2/1, AND1/2, NOT3/1
  [D] -> AND3/3, NOT4/1
  NOT2/1 -> AND1/1, AND/1
  NOT4/1 -> AND2/2, AND/2
  From11/1 -> OR3/1
  AND/1 -> OR3/3
  AND1/1 -> OR3/2
  AND2/1 -> OR3/4
  AND3/1 -> OR3/5
  OR3/1 -> d/1
  NOT3/1 -> AND3/2
  [D] -> NOT6/1
  NOT6/1 -> AND5/2, AND4/2
  NOT5/1 -> AND4/1
  [B] -> NOT5/1
  [C] -> AND5/1
  AND4/1 -> OR4/1
  AND5/1 -> OR4/2
  OR4/1 -> e/1
  [C] -> NOT7/1
  [D] -> NOT8/1
  NOT7/1 -> AND6/1, AND8/2
  NOT8/1 -> AND7/2, AND6/2
  [B] -> AND8/1, AND7/1
  From17/1 -> OR5/2
  AND6/1 -> OR5/1
  AND7/1 -> OR5/3
  AND8/1 -> OR5/4
  OR5/1 -> f/1
  [B] -> AND9/1, NOT10/1
  [C] -> AND11/2, AND10/1, NOT11/1
  [D] -> NOT12/1
  NOT11/1 -> AND9/2
  NOT12/1 -> AND10/2
  NOT10/1 -> AND11/1
  From21/1 -> OR6/1
  AND9/1 -> OR6/3
  AND10/1 -> OR6/2
  AND11/1 -> OR6/4
  OR6/1 -> g/1
  NOT13/1 -> OR/1
  NOT14/1 -> OR1/2

== system Clock_Model/CLOCK CIRCUIT/HOURS/MOD 13/MOD 10/Subsystem1 ==
  J : Inport
  K : Inport  Port=2
  CLK : Inport  Port=3
  CLR : Inport  Port=4
  Constant : Constant  Value=0
  Constant1 : Constant
  Data Type Conversion : DataTypeConversion  OutDataTypeStr=double  SaturateOnIntegerOverflow=off  RndMeth=Floor
  Data Type Conversion{1,3..5} (4 alike) : DataTypeConversion  OutDataTypeStr=boolean  SaturateOnIntegerOverflow=off  RndMeth=Floor
  Data Type Conversion2 : DataTypeConversion  OutDataTypeStr=double  SaturateOnIntegerOverflow=off  RndMeth=Floor
  J-K Flip-Flop : simulink_extras/Flip Flops/J-K Flip-Flop  initial_condition=0
  Memory : Memory
  Switch : Switch  Criteria=u2 > Threshold  Threshold=0.5  SaturateOnIntegerOverflow=off  InputSameDT=off
  Switch1 : Switch  Criteria=u2 > Threshold  Threshold=0.5  SaturateOnIntegerOverflow=off  InputSameDT=off
  Q : Outport
  Q BAR : Outport  Port=2
  wires:
  J-K Flip-Flop/1 -> Data Type Conversion4/1
  J-K Flip-Flop/2 -> Data Type Conversion5/1
  J/1 -> Data Type Conversion/1
  CLR/1 -> Memory/1
  [CLR] -> Switch/2
  Switch/1 -> Data Type Conversion1/1
  Data Type Conversion1/1 -> J-K Flip-Flop/1
  CLK/1 -> J-K Flip-Flop/2
  Data Type Conversion3/1 -> J-K Flip-Flop/3
  Switch1/1 -> Data Type Conversion3/1
  [CLR] -> Switch1/2
  K/1 -> Data Type Conversion2/1
  Memory/1 -> [CLR]
  Constant/1 -> Switch/1
  Data Type Conversion/1 -> Switch/3
  Data Type Conversion4/1 -> Q/1
  Data Type Conversion5/1 -> Q BAR/1
  Constant1/1 -> Switch1/1
  Data Type Conversion2/1 -> Switch1/3

== system Clock_Model/CLOCK CIRCUIT/HOURS/MOD 13/MOD 10/Subsystem2 ==
  J : Inport
  K : Inport  Port=2
  CLK : Inport  Port=3
  CLR : Inport  Port=4
  Constant : Constant  Value=0
  Constant1 : Constant
  Data Type Conversion : DataTypeConversion  OutDataTypeStr=double  SaturateOnIntegerOverflow=off  RndMeth=Floor
  Data Type Conversion{1,3..5} (4 alike) : DataTypeConversion  OutDataTypeStr=boolean  SaturateOnIntegerOverflow=off  RndMeth=Floor
  Data Type Conversion2 : DataTypeConversion  OutDataTypeStr=double  SaturateOnIntegerOverflow=off  RndMeth=Floor
  J-K Flip-Flop : simulink_extras/Flip Flops/J-K Flip-Flop  initial_condition=0
  Switch : Switch  Criteria=u2 > Threshold  Threshold=0.5  SaturateOnIntegerOverflow=off  InputSameDT=off
  Switch1 : Switch  Criteria=u2 > Threshold  Threshold=0.5  SaturateOnIntegerOverflow=off  InputSameDT=off
  Q : Outport
  Q BAR : Outport  Port=2
  wires:
  J-K Flip-Flop/1 -> Data Type Conversion4/1
  J-K Flip-Flop/2 -> Data Type Conversion5/1
  J/1 -> Data Type Conversion/1
  CLR/1 -> [CLR]
  [CLR] -> Switch/2
  Switch/1 -> Data Type Conversion1/1
  Data Type Conversion1/1 -> J-K Flip-Flop/1
  CLK/1 -> J-K Flip-Flop/2
  Data Type Conversion3/1 -> J-K Flip-Flop/3
  Switch1/1 -> Data Type Conversion3/1
  [CLR] -> Switch1/2
  K/1 -> Data Type Conversion2/1
  Constant/1 -> Switch/1
  Data Type Conversion/1 -> Switch/3
  Data Type Conversion4/1 -> Q/1
  Data Type Conversion5/1 -> Q BAR/1
  Constant1/1 -> Switch1/1
  Data Type Conversion2/1 -> Switch1/3

== system Clock_Model/CLOCK CIRCUIT/HOURS/MOD 13/MOD 10/Subsystem3 ==
  J : Inport
  K : Inport  Port=2
  CLK : Inport  Port=3
  CLR : Inport  Port=4
  Constant : Constant  Value=0
  Constant1 : Constant
  Data Type Conversion : DataTypeConversion  OutDataTypeStr=double  SaturateOnIntegerOverflow=off  RndMeth=Floor
  Data Type Conversion{1,3..5} (4 alike) : DataTypeConversion  OutDataTypeStr=boolean  SaturateOnIntegerOverflow=off  RndMeth=Floor
  Data Type Conversion2 : DataTypeConversion  OutDataTypeStr=double  SaturateOnIntegerOverflow=off  RndMeth=Floor
  J-K Flip-Flop : simulink_extras/Flip Flops/J-K Flip-Flop  initial_condition=0
  Switch : Switch  Criteria=u2 > Threshold  Threshold=0.5  SaturateOnIntegerOverflow=off  InputSameDT=off
  Switch1 : Switch  Criteria=u2 > Threshold  Threshold=0.5  SaturateOnIntegerOverflow=off  InputSameDT=off
  Q : Outport
  Q BAR : Outport  Port=2
  wires:
  J-K Flip-Flop/1 -> Data Type Conversion4/1
  J-K Flip-Flop/2 -> Data Type Conversion5/1
  J/1 -> Data Type Conversion/1
  CLR/1 -> [CLR]
  [CLR] -> Switch/2
  Switch/1 -> Data Type Conversion1/1
  Data Type Conversion1/1 -> J-K Flip-Flop/1
  CLK/1 -> J-K Flip-Flop/2
  Data Type Conversion3/1 -> J-K Flip-Flop/3
  Switch1/1 -> Data Type Conversion3/1
  [CLR] -> Switch1/2
  K/1 -> Data Type Conversion2/1
  Constant/1 -> Switch/1
  Data Type Conversion/1 -> Switch/3
  Data Type Conversion4/1 -> Q/1
  Data Type Conversion5/1 -> Q BAR/1
  Data Type Conversion2/1 -> Switch1/3
  Constant1/1 -> Switch1/1

== system Clock_Model/CLOCK CIRCUIT/HOURS/MOD 13/MOD 10/Subsystem4 ==
  J : Inport
  K : Inport  Port=2
  CLK : Inport  Port=3
  CLR : Inport  Port=4
  Constant : Constant  Value=0
  Constant1 : Constant
  Data Type Conversion : DataTypeConversion  OutDataTypeStr=double  SaturateOnIntegerOverflow=off  RndMeth=Floor
  Data Type Conversion{1,3..5} (4 alike) : DataTypeConversion  OutDataTypeStr=boolean  SaturateOnIntegerOverflow=off  RndMeth=Floor
  Data Type Conversion2 : DataTypeConversion  OutDataTypeStr=double  SaturateOnIntegerOverflow=off  RndMeth=Floor
  J-K Flip-Flop : simulink_extras/Flip Flops/J-K Flip-Flop  initial_condition=0
  Switch : Switch  Criteria=u2 > Threshold  Threshold=0.5  SaturateOnIntegerOverflow=off  InputSameDT=off
  Switch1 : Switch  Criteria=u2 > Threshold  Threshold=0.5  SaturateOnIntegerOverflow=off  InputSameDT=off
  Q : Outport
  Q BAR : Outport  Port=2
  wires:
  J-K Flip-Flop/1 -> Data Type Conversion4/1
  J-K Flip-Flop/2 -> Data Type Conversion5/1
  J/1 -> Data Type Conversion/1
  CLR/1 -> [CLR]
  [CLR] -> Switch/2
  Switch/1 -> Data Type Conversion1/1
  Data Type Conversion1/1 -> J-K Flip-Flop/1
  CLK/1 -> J-K Flip-Flop/2
  Data Type Conversion3/1 -> J-K Flip-Flop/3
  Switch1/1 -> Data Type Conversion3/1
  [CLR] -> Switch1/2
  K/1 -> Data Type Conversion2/1
  Data Type Conversion/1 -> Switch/3
  Constant/1 -> Switch/1
  Data Type Conversion4/1 -> Q/1
  Data Type Conversion5/1 -> Q BAR/1
  Constant1/1 -> Switch1/1
  Data Type Conversion2/1 -> Switch1/3

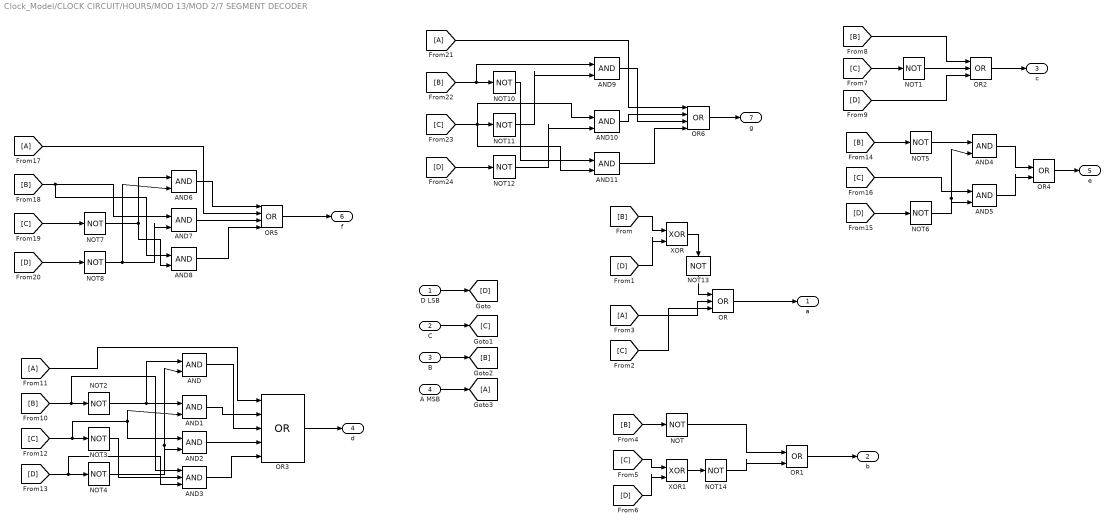
== system Clock_Model/CLOCK CIRCUIT/HOURS/MOD 13/MOD 2/7 SEGMENT DECODER ==
  D LSB : Inport
  C : Inport  Port=2
  B : Inport  Port=3
  A MSB : Inport  Port=4
  AND{,1..2,4..11} (11 alike) : Logic  IconShape=distinctive  AllPortsSameDT=off  OutDataTypeStr=boolean
  AND3 : Logic  Inputs=3  IconShape=distinctive  AllPortsSameDT=off  OutDataTypeStr=boolean
  From{3,11,17,21} (4 alike) : From
  Goto3 : Goto
  NOT{,1..8,10..14} (14 alike) : Logic  Operator=NOT  IconShape=distinctive  AllPortsSameDT=off  OutDataTypeStr=boolean
  OR : Logic  Operator=OR  Inputs=3  IconShape=distinctive  AllPortsSameDT=off  OutDataTypeStr=boolean
  OR1 : Logic  Operator=OR  IconShape=distinctive  AllPortsSameDT=off  OutDataTypeStr=boolean
  OR2 : Logic  Operator=OR  Inputs=3  IconShape=distinctive  AllPortsSameDT=off  OutDataTypeStr=boolean
  OR3 : Logic  Operator=OR  Inputs=5  IconShape=distinctive  AllPortsSameDT=off  OutDataTypeStr=boolean
  OR4 : Logic  Operator=OR  IconShape=distinctive  AllPortsSameDT=off  OutDataTypeStr=boolean
  OR5 : Logic  Operator=OR  Inputs=4  IconShape=distinctive  AllPortsSameDT=off  OutDataTypeStr=boolean
  OR6 : Logic  Operator=OR  Inputs=4  IconShape=distinctive  AllPortsSameDT=off  OutDataTypeStr=boolean
  XOR : Logic  Operator=XOR  IconShape=distinctive  AllPortsSameDT=off  OutDataTypeStr=boolean
  XOR1 : Logic  Operator=XOR  IconShape=distinctive  AllPortsSameDT=off  OutDataTypeStr=boolean
  a : Outport
  b : Outport  Port=2
  c : Outport  Port=3
  d : Outport  Port=4
  e : Outport  Port=5
  f : Outport  Port=6
  g : Outport  Port=7
  wires:
  D LSB/1 -> [D]
  C/1 -> [C]
  B/1 -> [B]
  A MSB/1 -> Goto3/1
  XOR/1 -> NOT13/1
  [B] -> XOR/1
  [D] -> XOR/2
  From3/1 -> OR/2
  [C] -> OR/3
  OR/1 -> a/1
  [B] -> NOT/1
  [C] -> XOR1/1
  [D] -> XOR1/2
  NOT/1 -> OR1/1
  XOR1/1 -> NOT14/1
  OR1/1 -> b/1
  [C] -> NOT1/1
  [B] -> OR2/1
  NOT1/1 -> OR2/2
  [D] -> OR2/3
  OR2/1 -> c/1
  [B] -> AND3/1, NOT2/1
  [C] -> AND2/1, AND1/2, NOT3/1
  [D] -> AND3/3, NOT4/1
  NOT2/1 -> AND1/1, AND/1
  NOT4/1 -> AND2/2, AND/2
  From11/1 -> OR3/1
  AND/1 -> OR3/3
  AND1/1 -> OR3/2
  AND2/1 -> OR3/4
  AND3/1 -> OR3/5
  OR3/1 -> d/1
  NOT3/1 -> AND3/2
  [D] -> NOT6/1
  NOT6/1 -> AND5/2, AND4/2
  NOT5/1 -> AND4/1
  [B] -> NOT5/1
  [C] -> AND5/1
  AND4/1 -> OR4/1
  AND5/1 -> OR4/2
  OR4/1 -> e/1
  [C] -> NOT7/1
  [D] -> NOT8/1
  NOT7/1 -> AND6/1, AND8/2
  NOT8/1 -> AND7/2, AND6/2
  [B] -> AND8/1, AND7/1
  From17/1 -> OR5/2
  AND6/1 -> OR5/1
  AND7/1 -> OR5/3
  AND8/1 -> OR5/4
  OR5/1 -> f/1
  [B] -> AND9/1, NOT10/1
  [C] -> AND11/2, AND10/1, NOT11/1
  [D] -> NOT12/1
  NOT11/1 -> AND9/2
  NOT12/1 -> AND10/2
  NOT10/1 -> AND11/1
  From21/1 -> OR6/1
  AND9/1 -> OR6/3
  AND10/1 -> OR6/2
  AND11/1 -> OR6/4
  OR6/1 -> g/1
  NOT13/1 -> OR/1
  NOT14/1 -> OR1/2

== system Clock_Model/CLOCK CIRCUIT/HOURS/MOD 13/MOD 2/Subsystem1 ==
  J : Inport
  K : Inport  Port=2
  CLK : Inport  Port=3
  CLR : Inport  Port=4
  Constant : Constant  Value=0
  Constant1 : Constant
  Data Type Conversion : DataTypeConversion  OutDataTypeStr=double  SaturateOnIntegerOverflow=off  RndMeth=Floor
  Data Type Conversion{1,3..5} (4 alike) : DataTypeConversion  OutDataTypeStr=boolean  SaturateOnIntegerOverflow=off  RndMeth=Floor
  Data Type Conversion2 : DataTypeConversion  OutDataTypeStr=double  SaturateOnIntegerOverflow=off  RndMeth=Floor
  J-K Flip-Flop : simulink_extras/Flip Flops/J-K Flip-Flop  initial_condition=0
  Memory : Memory
  Switch : Switch  Criteria=u2 > Threshold  Threshold=0.5  SaturateOnIntegerOverflow=off  InputSameDT=off
  Switch1 : Switch  Criteria=u2 > Threshold  Threshold=0.5  SaturateOnIntegerOverflow=off  InputSameDT=off
  Q : Outport
  Q BAR : Outport  Port=2
  wires:
  J-K Flip-Flop/1 -> Data Type Conversion4/1
  J-K Flip-Flop/2 -> Data Type Conversion5/1
  J/1 -> Data Type Conversion/1
  CLR/1 -> Memory/1
  [CLR] -> Switch/2
  Switch/1 -> Data Type Conversion1/1
  Data Type Conversion1/1 -> J-K Flip-Flop/1
  CLK/1 -> J-K Flip-Flop/2
  Data Type Conversion3/1 -> J-K Flip-Flop/3
  Switch1/1 -> Data Type Conversion3/1
  [CLR] -> Switch1/2
  K/1 -> Data Type Conversion2/1
  Memory/1 -> [CLR]
  Constant/1 -> Switch/1
  Data Type Conversion/1 -> Switch/3
  Data Type Conversion4/1 -> Q/1
  Data Type Conversion5/1 -> Q BAR/1
  Constant1/1 -> Switch1/1
  Data Type Conversion2/1 -> Switch1/3

== system Clock_Model/CLOCK CIRCUIT/HOURS/MOD 13/MOD 2/Subsystem2 ==
  J : Inport
  K : Inport  Port=2
  CLK : Inport  Port=3
  CLR : Inport  Port=4
  Constant : Constant  Value=0
  Constant1 : Constant
  Data Type Conversion : DataTypeConversion  OutDataTypeStr=double  SaturateOnIntegerOverflow=off  RndMeth=Floor
  Data Type Conversion{1,3..5} (4 alike) : DataTypeConversion  OutDataTypeStr=boolean  SaturateOnIntegerOverflow=off  RndMeth=Floor
  Data Type Conversion2 : DataTypeConversion  OutDataTypeStr=double  SaturateOnIntegerOverflow=off  RndMeth=Floor
  J-K Flip-Flop : simulink_extras/Flip Flops/J-K Flip-Flop  initial_condition=0
  Switch : Switch  Criteria=u2 > Threshold  Threshold=0.5  SaturateOnIntegerOverflow=off  InputSameDT=off
  Switch1 : Switch  Criteria=u2 > Threshold  Threshold=0.5  SaturateOnIntegerOverflow=off  InputSameDT=off
  Q : Outport
  Q BAR : Outport  Port=2
  wires:
  J-K Flip-Flop/1 -> Data Type Conversion4/1
  J-K Flip-Flop/2 -> Data Type Conversion5/1
  J/1 -> Data Type Conversion/1
  CLR/1 -> [CLR]
  [CLR] -> Switch/2
  Switch/1 -> Data Type Conversion1/1
  Data Type Conversion1/1 -> J-K Flip-Flop/1
  CLK/1 -> J-K Flip-Flop/2
  Data Type Conversion3/1 -> J-K Flip-Flop/3
  Switch1/1 -> Data Type Conversion3/1
  [CLR] -> Switch1/2
  K/1 -> Data Type Conversion2/1
  Constant/1 -> Switch/1
  Data Type Conversion/1 -> Switch/3
  Data Type Conversion4/1 -> Q/1
  Data Type Conversion5/1 -> Q BAR/1
  Constant1/1 -> Switch1/1
  Data Type Conversion2/1 -> Switch1/3

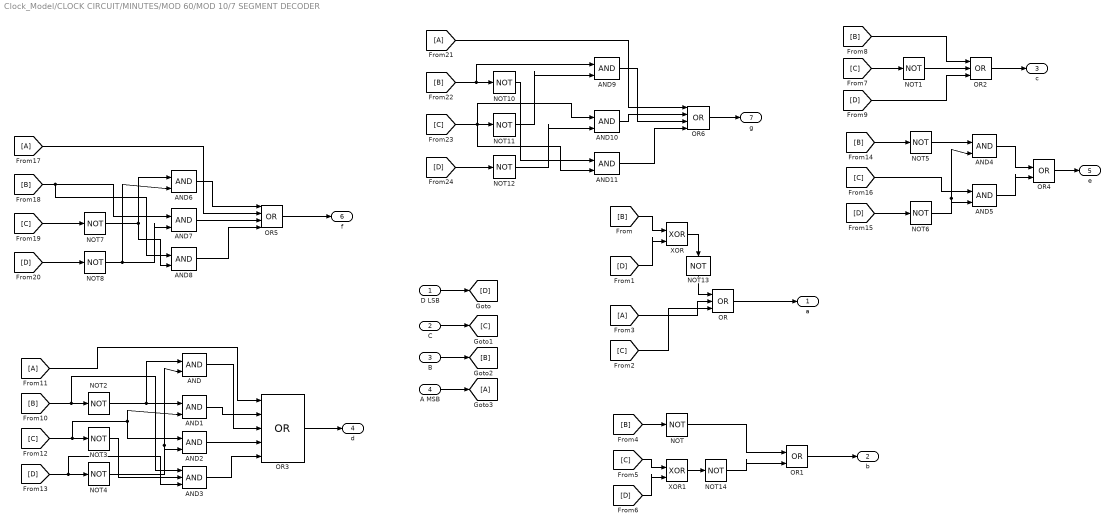
== system Clock_Model/CLOCK CIRCUIT/MINUTES/MOD 60/MOD 10/7 SEGMENT DECODER ==
  D LSB : Inport
  C : Inport  Port=2
  B : Inport  Port=3
  A MSB : Inport  Port=4
  AND{,1..2,4..11} (11 alike) : Logic  IconShape=distinctive  AllPortsSameDT=off  OutDataTypeStr=boolean
  AND3 : Logic  Inputs=3  IconShape=distinctive  AllPortsSameDT=off  OutDataTypeStr=boolean
  From{3,11,17,21} (4 alike) : From
  Goto3 : Goto
  NOT{,1..8,10..14} (14 alike) : Logic  Operator=NOT  IconShape=distinctive  AllPortsSameDT=off  OutDataTypeStr=boolean
  OR : Logic  Operator=OR  Inputs=3  IconShape=distinctive  AllPortsSameDT=off  OutDataTypeStr=boolean
  OR1 : Logic  Operator=OR  IconShape=distinctive  AllPortsSameDT=off  OutDataTypeStr=boolean
  OR2 : Logic  Operator=OR  Inputs=3  IconShape=distinctive  AllPortsSameDT=off  OutDataTypeStr=boolean
  OR3 : Logic  Operator=OR  Inputs=5  IconShape=distinctive  AllPortsSameDT=off  OutDataTypeStr=boolean
  OR4 : Logic  Operator=OR  IconShape=distinctive  AllPortsSameDT=off  OutDataTypeStr=boolean
  OR5 : Logic  Operator=OR  Inputs=4  IconShape=distinctive  AllPortsSameDT=off  OutDataTypeStr=boolean
  OR6 : Logic  Operator=OR  Inputs=4  IconShape=distinctive  AllPortsSameDT=off  OutDataTypeStr=boolean
  XOR : Logic  Operator=XOR  IconShape=distinctive  AllPortsSameDT=off  OutDataTypeStr=boolean
  XOR1 : Logic  Operator=XOR  IconShape=distinctive  AllPortsSameDT=off  OutDataTypeStr=boolean
  a : Outport
  b : Outport  Port=2
  c : Outport  Port=3
  d : Outport  Port=4
  e : Outport  Port=5
  f : Outport  Port=6
  g : Outport  Port=7
  wires:
  D LSB/1 -> [D]
  C/1 -> [C]
  B/1 -> [B]
  A MSB/1 -> Goto3/1
  XOR/1 -> NOT13/1
  [B] -> XOR/1
  [D] -> XOR/2
  From3/1 -> OR/2
  [C] -> OR/3
  OR/1 -> a/1
  [B] -> NOT/1
  [C] -> XOR1/1
  [D] -> XOR1/2
  NOT/1 -> OR1/1
  XOR1/1 -> NOT14/1
  OR1/1 -> b/1
  [C] -> NOT1/1
  [B] -> OR2/1
  NOT1/1 -> OR2/2
  [D] -> OR2/3
  OR2/1 -> c/1
  [B] -> AND3/1, NOT2/1
  [C] -> AND2/1, AND1/2, NOT3/1
  [D] -> AND3/3, NOT4/1
  NOT2/1 -> AND1/1, AND/1
  NOT4/1 -> AND2/2, AND/2
  From11/1 -> OR3/1
  AND/1 -> OR3/3
  AND1/1 -> OR3/2
  AND2/1 -> OR3/4
  AND3/1 -> OR3/5
  OR3/1 -> d/1
  NOT3/1 -> AND3/2
  [D] -> NOT6/1
  NOT6/1 -> AND5/2, AND4/2
  NOT5/1 -> AND4/1
  [B] -> NOT5/1
  [C] -> AND5/1
  AND4/1 -> OR4/1
  AND5/1 -> OR4/2
  OR4/1 -> e/1
  [C] -> NOT7/1
  [D] -> NOT8/1
  NOT7/1 -> AND6/1, AND8/2
  NOT8/1 -> AND7/2, AND6/2
  [B] -> AND8/1, AND7/1
  From17/1 -> OR5/2
  AND6/1 -> OR5/1
  AND7/1 -> OR5/3
  AND8/1 -> OR5/4
  OR5/1 -> f/1
  [B] -> AND9/1, NOT10/1
  [C] -> AND11/2, AND10/1, NOT11/1
  [D] -> NOT12/1
  NOT11/1 -> AND9/2
  NOT12/1 -> AND10/2
  NOT10/1 -> AND11/1
  From21/1 -> OR6/1
  AND9/1 -> OR6/3
  AND10/1 -> OR6/2
  AND11/1 -> OR6/4
  OR6/1 -> g/1
  NOT13/1 -> OR/1
  NOT14/1 -> OR1/2

== system Clock_Model/CLOCK CIRCUIT/MINUTES/MOD 60/MOD 10/Subsystem1 ==
  J : Inport
  K : Inport  Port=2
  CLK : Inport  Port=3
  CLR : Inport  Port=4
  Constant : Constant  Value=0
  Constant1 : Constant
  Data Type Conversion : DataTypeConversion  OutDataTypeStr=double  SaturateOnIntegerOverflow=off  RndMeth=Floor
  Data Type Conversion{1,3..5} (4 alike) : DataTypeConversion  OutDataTypeStr=boolean  SaturateOnIntegerOverflow=off  RndMeth=Floor
  Data Type Conversion2 : DataTypeConversion  OutDataTypeStr=double  SaturateOnIntegerOverflow=off  RndMeth=Floor
  J-K Flip-Flop : simulink_extras/Flip Flops/J-K Flip-Flop  initial_condition=0
  Memory : Memory
  Switch : Switch  Criteria=u2 > Threshold  Threshold=0.5  SaturateOnIntegerOverflow=off  InputSameDT=off
  Switch1 : Switch  Criteria=u2 > Threshold  Threshold=0.5  SaturateOnIntegerOverflow=off  InputSameDT=off
  Q : Outport
  Q BAR : Outport  Port=2
  wires:
  J-K Flip-Flop/1 -> Data Type Conversion4/1
  J-K Flip-Flop/2 -> Data Type Conversion5/1
  J/1 -> Data Type Conversion/1
  CLR/1 -> Memory/1
  [CLR] -> Switch/2
  Switch/1 -> Data Type Conversion1/1
  Data Type Conversion1/1 -> J-K Flip-Flop/1
  CLK/1 -> J-K Flip-Flop/2
  Data Type Conversion3/1 -> J-K Flip-Flop/3
  Switch1/1 -> Data Type Conversion3/1
  [CLR] -> Switch1/2
  K/1 -> Data Type Conversion2/1
  Memory/1 -> [CLR]
  Constant/1 -> Switch/1
  Data Type Conversion/1 -> Switch/3
  Data Type Conversion4/1 -> Q/1
  Data Type Conversion5/1 -> Q BAR/1
  Constant1/1 -> Switch1/1
  Data Type Conversion2/1 -> Switch1/3

== system Clock_Model/CLOCK CIRCUIT/MINUTES/MOD 60/MOD 10/Subsystem2 ==
  J : Inport
  K : Inport  Port=2
  CLK : Inport  Port=3
  CLR : Inport  Port=4
  Constant : Constant  Value=0
  Constant1 : Constant
  Data Type Conversion : DataTypeConversion  OutDataTypeStr=double  SaturateOnIntegerOverflow=off  RndMeth=Floor
  Data Type Conversion{1,3..5} (4 alike) : DataTypeConversion  OutDataTypeStr=boolean  SaturateOnIntegerOverflow=off  RndMeth=Floor
  Data Type Conversion2 : DataTypeConversion  OutDataTypeStr=double  SaturateOnIntegerOverflow=off  RndMeth=Floor
  J-K Flip-Flop : simulink_extras/Flip Flops/J-K Flip-Flop  initial_condition=0
  Switch : Switch  Criteria=u2 > Threshold  Threshold=0.5  SaturateOnIntegerOverflow=off  InputSameDT=off
  Switch1 : Switch  Criteria=u2 > Threshold  Threshold=0.5  SaturateOnIntegerOverflow=off  InputSameDT=off
  Q : Outport
  Q BAR : Outport  Port=2
  wires:
  J-K Flip-Flop/1 -> Data Type Conversion4/1
  J-K Flip-Flop/2 -> Data Type Conversion5/1
  J/1 -> Data Type Conversion/1
  CLR/1 -> [CLR]
  [CLR] -> Switch/2
  Switch/1 -> Data Type Conversion1/1
  Data Type Conversion1/1 -> J-K Flip-Flop/1
  CLK/1 -> J-K Flip-Flop/2
  Data Type Conversion3/1 -> J-K Flip-Flop/3
  Switch1/1 -> Data Type Conversion3/1
  [CLR] -> Switch1/2
  K/1 -> Data Type Conversion2/1
  Constant/1 -> Switch/1
  Data Type Conversion/1 -> Switch/3
  Data Type Conversion4/1 -> Q/1
  Data Type Conversion5/1 -> Q BAR/1
  Constant1/1 -> Switch1/1
  Data Type Conversion2/1 -> Switch1/3

== system Clock_Model/CLOCK CIRCUIT/MINUTES/MOD 60/MOD 10/Subsystem3 ==
  J : Inport
  K : Inport  Port=2
  CLK : Inport  Port=3
  CLR : Inport  Port=4
  Constant : Constant  Value=0
  Constant1 : Constant
  Data Type Conversion : DataTypeConversion  OutDataTypeStr=double  SaturateOnIntegerOverflow=off  RndMeth=Floor
  Data Type Conversion{1,3..5} (4 alike) : DataTypeConversion  OutDataTypeStr=boolean  SaturateOnIntegerOverflow=off  RndMeth=Floor
  Data Type Conversion2 : DataTypeConversion  OutDataTypeStr=double  SaturateOnIntegerOverflow=off  RndMeth=Floor
  J-K Flip-Flop : simulink_extras/Flip Flops/J-K Flip-Flop  initial_condition=0
  Switch : Switch  Criteria=u2 > Threshold  Threshold=0.5  SaturateOnIntegerOverflow=off  InputSameDT=off
  Switch1 : Switch  Criteria=u2 > Threshold  Threshold=0.5  SaturateOnIntegerOverflow=off  InputSameDT=off
  Q : Outport
  Q BAR : Outport  Port=2
  wires:
  J-K Flip-Flop/1 -> Data Type Conversion4/1
  J-K Flip-Flop/2 -> Data Type Conversion5/1
  J/1 -> Data Type Conversion/1
  CLR/1 -> [CLR]
  [CLR] -> Switch/2
  Switch/1 -> Data Type Conversion1/1
  Data Type Conversion1/1 -> J-K Flip-Flop/1
  CLK/1 -> J-K Flip-Flop/2
  Data Type Conversion3/1 -> J-K Flip-Flop/3
  Switch1/1 -> Data Type Conversion3/1
  [CLR] -> Switch1/2
  K/1 -> Data Type Conversion2/1
  Constant/1 -> Switch/1
  Data Type Conversion/1 -> Switch/3
  Data Type Conversion4/1 -> Q/1
  Data Type Conversion5/1 -> Q BAR/1
  Data Type Conversion2/1 -> Switch1/3
  Constant1/1 -> Switch1/1
